simulink model "zynqRadioWalkieTalkieTxAD9361AD9364SL"  (R2016a)
settings: Solver=ode45  StartTime=0.0  StopTime=inf  RelTol=1e-3
PostLoadFcn:
  | sdrzWalkieTalkieTxParams = zynqRadioWalkieTalkieTxHelperAD9361AD9364SL_SimParams;
  | sdrzWalkieTalkieTxHelper_ModelParamsMask('applyParametersToModel');
InitFcn:
  | sdrzWalkieTalkieTxParams = zynqRadioWalkieTalkieTxHelperAD9361AD9364SL_SimParams;
  | sdrzWalkieTalkieTxHelper_ModelParamsMask('applyParametersToModel');
libraries: dspsrcs4 x3, dspvision x1, sdrzblksprivate x1, zc706fmc234_lib x1, dspmlti4 x1
CloseFcn:
  | clear sdrzWalkieTalkieTxParams
Description:
  | This model uses Simulink(R) to transmit an FM signal suitable for reception on a commercial walkie-talkie using SDR hardware.
settings Model: SimulationMode=accelerator  Creator=The MathWorks, Inc.  LastModifiedBy=The MathWorks, Inc.
settings DataIOCC: LimitDataPoints=on  SaveFormat=Array
settings DebuggingCC: SolverPrmCheckMsg=warning  ParameterPrecisionLossMsg=none  AllowSymbolicDim=off
settings HardwareCC: ProdBitPerPointer=32  ProdLargestAtomicFloat=None  ProdIntDivRoundTo=Undefined  ProdEndianess=Unspecified  ProdWordSize=32  ProdHWDeviceType=32-bit Generic
settings ModelReferenceCC: PropagateSignalLabelsOutOfModel=off
settings ConfigComp: CovModelRefEnable=Off  CovSFcnEnable=off

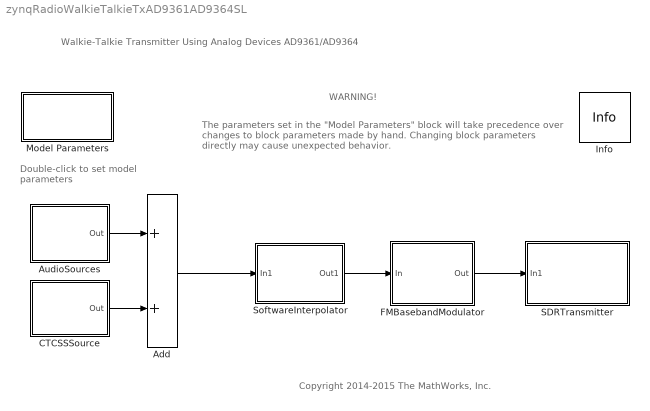
== system zynqRadioWalkieTalkieTxAD9361AD9364SL ==
  note: Walkie-Talkie Transmitter Using Analog Devices AD9361/AD9364
  note: Double-click to
      | set model parameters
  note: The parameters set in the "Model Parameters" block will
      | take precedence over changes to block parameters made by hand.
      | Changing block parameters directly may cause unexpected behavior.
  note: WARNING!
  note: Copyright 2014-2015 The MathWorks, Inc.
  Add : Sum
  AudioSources : Subsystem
      mask Display: fprintf('Audio\nGenerator');
  CTCSSSource : Subsystem
      mask Display: fprintf('CTCSS\nGenerator');
  FMBasebandModulator : Subsystem
      mask Display: disp('FM Baseband\nModulator');
  Info : sdrzblksprivate/Info  SystemSampleTime=-1
  Model Parameters : Subsystem  TreatAsAtomicUnit=on  SystemSampleTime=sdrzWalkieTalkieTxParams.audioSampleRate  mask(Model Parameters){audioSource=Sound file, toneFrequency=880, targetSweepTime=3, normalizedTransmitPower=0.9, walkieTalkieProtocol=FRS, channelFRS=1, channelPMR446=3, CTCSSCode=5, CTCSSAmplitude=0.15}
      mask prompts: audioSource "Signal selection:"; toneFrequency "Pure tone frequency (Hz):"; targetSweepTime "Chirp target/sweep time (s):"; normalizedTransmitPower "Normalized transmit power:"; walkieTalkieProtocol "Walkie-talkie protocol:"; channelFRS "Channel (1 to 14):"; channelPMR446 "Channel (1 to 8):"; CTCSSCode "CTCSS code (1 to 38):"; CTCSSAmplitude "Normalized CTCSS amplitude:"
      mask help: Changing these values defines the model parameters needed for a transmission.
      mask init:
      | sdrzWalkieTalkieTxHelper_ModelParamsMask('applyParametersToModel');
      mask Help: sdrzdemohelp;
      mask TypeOptions audioSource: Pure tone | Chirp | Sound file
      mask Callback audioSource: sdrzWalkieTalkieTxHelper_ModelParamsMask('maskDisplayUpdate');
      mask TypeOptions walkieTalkieProtocol: FRS | PMR446
      mask Callback walkieTalkieProtocol: sdrzWalkieTalkieTxHelper_ModelParamsMask('maskDisplayUpdate');
      mask Display: disp('Model\nParameters');
  SDRTransmitter : Subsystem
      mask Display: fprintf('SDR\nTransmitter')
  SoftwareInterpolator : Subsystem
      mask Display: fprintf('Software\nInterpolator')
  wires:
  CTCSSSource/1(Out) -> Add/2
  AudioSources/1(Out) -> Add/1
  Add/1 -> SoftwareInterpolator/1(In1)
  SoftwareInterpolator/1(Out1) -> FMBasebandModulator/1(In)
  FMBasebandModulator/1(Out) -> SDRTransmitter/1(In1)

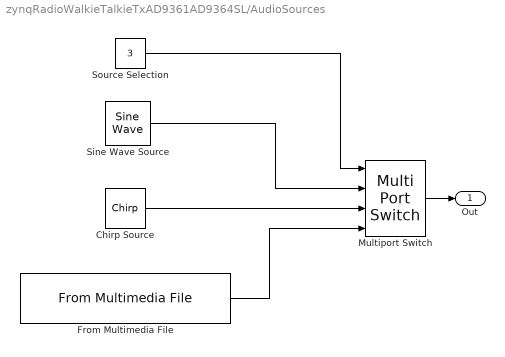
== system zynqRadioWalkieTalkieTxAD9361AD9364SL/AudioSources ==
  Chirp Source : dspsrcs4/Chirp  sweep=Linear  mode=Unidirectional  f0=500  f1=3400  t1=3  Tsweep=3  phase=0  Ts=sdrzWalkieTalkieTxParams.audioSamplePeriod  spf=sdrzWalkieTalkieTxParams.audioFrameSize  datatype=Single  OutputFrames=off
  From Multimedia File : dspvision/From Multimedia File  inputFilename=sdrzWalkieTalkieHelper_voice.wav  loop=on  numPlays=inf  outputStreams=Audio only  videoDataType=single  audioDataType=single  inheritSampleTime=on  userDefinedSampleTime=1/30  noAudioOutput=off  isIntensityVideo=off  fourcc=RGB  colorVideoFormat=Separate color signals  outputEOF=off  dataOrg=Column-major  audioFrameSize=sdrzWalkieTalkieTxParams.audioFrameSize  computeAudioFrameSize=off  outSamplingMode=Sample based
  Multiport Switch : MultiPortSwitch
  Sine Wave Source : dspsrcs4/Sine Wave  Amplitude=1  Frequency=880  Phase=0  SampleMode=Discrete  OutComplex=Real  CompMethod=Trigonometric fcn  TableSize=Speed  SampleTime=sdrzWalkieTalkieTxParams.audioSamplePeriod  SamplesPerFrame=sdrzWalkieTalkieTxParams.audioFrameSize  ResetState=Restart at time zero  OutputFrames=off  dataType=single  wordLen=16  udDataType=sfix(16)  fracBitsMode=Best precision  numFracBits=15  OutDataTypeStr=single  LastOutDataTypeStr=single
  Source Selection : Constant  Tag=SourceSelection  Value=3
  Out : Outport
  wires:
  Multiport Switch/1 -> Out/1
  Source Selection/1 -> Multiport Switch/1
  Chirp Source/1 -> Multiport Switch/3
  Sine Wave Source/1 -> Multiport Switch/2
  From Multimedia File/1 -> Multiport Switch/4

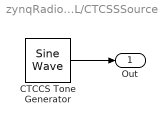
== system zynqRadioWalkieTalkieTxAD9361AD9364SL/CTCSSSource ==
  CTCCS Tone Generator : dspsrcs4/Sine Wave  Amplitude=0.15  Frequency=79.7  Phase=0  SampleMode=Discrete  OutComplex=Real  CompMethod=Trigonometric fcn  TableSize=Speed  SampleTime=sdrzWalkieTalkieTxParams.audioSamplePeriod  SamplesPerFrame=sdrzWalkieTalkieTxParams.audioFrameSize  ResetState=Restart at time zero  OutputFrames=off  dataType=single  wordLen=16  udDataType=sfix(16)  fracBitsMode=Best precision  numFracBits=15  OutDataTypeStr=single  LastOutDataTypeStr=single
  Out : Outport
  wires:
  CTCCS Tone Generator/1 -> Out/1

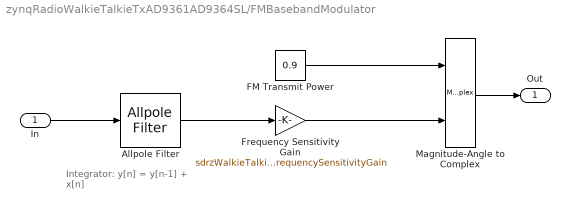
== system zynqRadioWalkieTalkieTxAD9361AD9364SL/FMBasebandModulator ==
  note: Integrator:
      | y[n] = y[n-1] + x[n]
  In : Inport
  Allpole Filter : AllpoleFilter  FilterStructure=Direct form transposed  Coefficients=[1 -1]  AccumDataTypeStr=Inherit: Same as product output  OutDataTypeStr=Inherit: Same as accumulator
  FM Transmit Power : Constant  Value=0.9  OutDataTypeStr=single
  Frequency Sensitivity Gain : Gain  Gain=sdrzWalkieTalkieTxParams.frequencySensitivityGain
  Magnitude-Angle to Complex : MagnitudeAngleToComplex
  Out : Outport
  wires:
  Frequency Sensitivity Gain/1 -> Magnitude-Angle to Complex/2
  Allpole Filter/1 -> Frequency Sensitivity Gain/1
  In/1 -> Allpole Filter/1
  Magnitude-Angle to Complex/1 -> Out/1
  FM Transmit Power/1 -> Magnitude-Angle to Complex/1

== system zynqRadioWalkieTalkieTxAD9361AD9364SL/Model Parameters ==
  note: This subsystem is empty.
      | It is used for setting parameter values (in the mask).

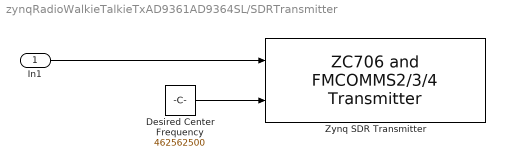
== system zynqRadioWalkieTalkieTxAD9361AD9364SL/SDRTransmitter ==
  In1 : Inport
  Desired Center Frequency : Constant  Value=462562500
  Zynq SDR Transmitter : zc706fmc234_lib/ZC706 and  FMCOMMS2//3//4  Transmitter  IPAddress=192.168.3.2  CenterFrequencySource=Input port  CenterFrequency=2400000000  GainSource=Dialog  Gain=-10  ChannelMapping=1  BasebandSampleRate=sdrzWalkieTalkieTxParams.radioSampleRate  EnableBurstMode=off  NumFramesInBurst=20  DMATimeoutValue=1  EnableTxPrimingMode=on  blockMode=Normal  LostSamplesOutputPort=off  OverflowOutputPort=off  DataSourceSelect=Host  DDSFrequency=[ 1000000, 1000000; 1000000, 1000000 ]  DDSPhase=[ 0, 0; 0, 0 ]  DDSScale=[ 250000, 250000; 250000, 250000 ]  BypassUserLogic=on  ShowAdvancedProperties=on  ShowInternalProperties=off  subDeviceList=zynqTransmitter  sdrExecutionMode=HW  dataUDPPort=-1  ctrlUDPPort=-1  FIRCoefficientSize=[ 128; 128 ]  FIRCoefficients=[ 111, -87, 147, -127, -18, -286, -312, -555, -601, -722, -642, -555, -303, -66, 221, 393, 488, 403, 219, -74, -343, -550, -582, -450, -146, 221, 569, 759, 735, 463, 20, -487, -885, -1048, -883, -418, 243, 897, 1340, 1394, 1002, 228, -715, -1549, -1980, -1819, -1028, 217, 1583, 2635, 2980, 2377, 853, -1275, -3435, -4926, -5080, -3454, 40, 5065, 10903, 16581, 21085, 23573, 23573, 21085, 16581, 10903, 5065, 40, -3454, -5080, -4926, -3435, -1275, 853, 2377, 2980, 2635, 1583, 217, -1028, -1819, -1980, -1549, -715, 228, 1002, 1394, 1340, 897, 243, -418, -883, -1048, -885, -487, 20, 463, 735, 759, 569, 221, -146, -450, -582, -550, -343, -74, 219, 403, 488, 393, 221, -66, -303, -555, -642, -722, -601, -555, -312, -286, -18, -127, 147, -87, 111; 382, -200, 711, -41, 645, 36, 346, -194, -119, -543, -472, -646, -404, -312, 45, 197, 413, 346, 241, -93, -373, -680, -755, -689, -356, 51, 515, 795, 870, 609, 136, -488, -1009, -1303, -1191, -712, 69, 885, 1516, 1692, 1336, 468, -662, -1740, -2378, -2329, -1494, -55, 1620, 2995, 3584, 3045, 1368, -1121, -3755, -5708, -6156, -4542, -710, 4969, 11669, 18243, 23486, 26391, 26391, 23486, 18243, 11669, 4969, -710, -4542, -6156, -5708, -3755, -1121, 1368, 3045, 3584, 2995, 1620, -55, -1494, -2329, -2378, -1740, -662, 468, 1336, 1692, 1516, 885, 69, -712, -1191, -1303, -1009, -488, 136, 609, 870, 795, 515, 51, -356, -689, -755, -680, -373, -93, 241, 346, 413, 197, 45, -312, -404, -646, -472, -543, -119, -194, 346, 36, 645, -41, 711, -200, 382 ]  FIRGain=[ 0; -12 ]  FIRDecimInterpFactor=[ 4; 4 ]  AnalogFilterCutoff=[ 2560000; 2560000 ]  FilterPathRates=[ 737280000, 184320000, 61440000, 30720000, 15360000, 3840000; 737280000, 184320000, 61440000, 30720000, 15360000, 3840000 ]  FilterDesignTypeForTx=DefaultFilter  FilterDesignTypeForRx=DefaultFilterFromOther  SimulateUsing=Code generation
  wires:
  Desired Center Frequency/1 -> Zynq SDR Transmitter/2
  In1/1 -> Zynq SDR Transmitter/1

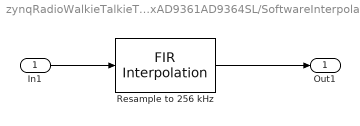
== system zynqRadioWalkieTalkieTxAD9361AD9364SL/SoftwareInterpolator ==
  In1 : Inport
  Resample to 256 kHz : dspmlti4/FIR Interpolation  FilterSource=Auto  h=sdrzWalkieTalkieTxParams.interpolatorCoefficients  L=sdrzWalkieTalkieTxParams.softwareInterpolationFactor  FilterObject=Hm_firinterp  InputProcessing=Columns as channels (frame based)  framing=Enforce single-rate processing  outputBufInitCond=0  roundingMode=Floor  overflowMode=off  firstCoeffDataTypeStr=Inherit: Same word length as input  firstCoeffMin=[]  firstCoeffMax=[]  firstCoeffLastDataTypeStr=Inherit: Same word length as input  outputDataTypeStr=Inherit: Same as accumulator  outputMin=[]  outputMax=[]  outputLastDataTypeStr=Inherit: Same as accumulator
  Out1 : Outport
  wires:
  Resample to 256 kHz/1 -> Out1/1
  In1/1 -> Resample to 256 kHz/1
